simulink model "Sensor_Model"  (R2017b)
settings: Solver=VariableStepAuto  StartTime=0.0  StopTime=10.0  RelTol=1e-3
libraries: aerolibatmos2 x2
settings Model: Creator=pc  LastModifiedBy=pc

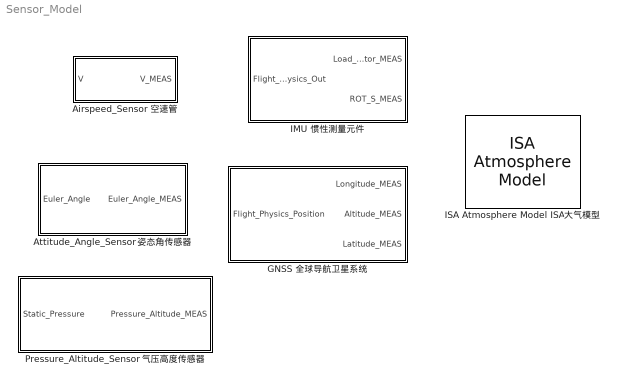
== system Sensor_Model ==
  Airspeed_Sensor 空速管 : Subsystem
  Attitude_Angle_Sensor 姿态角传感器 : Subsystem
  "GNSS 全球导航卫星系统 " : Subsystem
  IMU 惯性测量元件 : Subsystem
  ISA Atmosphere Model ISA大气模型 : aerolibatmos2/ISA Atmosphere Model  custom=off  g=9.80665  gamma=1.4  R=287.0531  L=0.0065  h_trop=11000  h_strat=20000  rho0=1.225  P0=101325  T0=288.15  h0=0
      settings: SourceProductName=Aerospace Blockset
  Pressure_Altitude_Sensor 气压高度传感器 : Subsystem

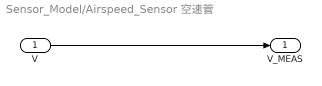
== system Sensor_Model/Airspeed_Sensor 空速管 ==
  V : Inport
  V_MEAS : Outport
  wires:
  V/1 -> V_MEAS/1

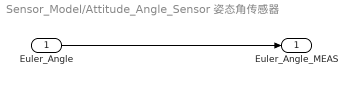
== system Sensor_Model/Attitude_Angle_Sensor 姿态角传感器 ==
  Euler_Angle : Inport
  Euler_Angle_MEAS : Outport
  wires:
  Euler_Angle/1 -> Euler_Angle_MEAS/1

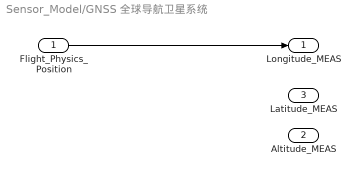
== system Sensor_Model/GNSS 全球导航卫星系统  ==
  Flight_Physics_Position : Inport
  Longitude_MEAS : Outport
  Altitude_MEAS : Outport  Port=2
  Latitude_MEAS : Outport  Port=3
  wires:
  Flight_Physics_Position/1 -> Longitude_MEAS/1

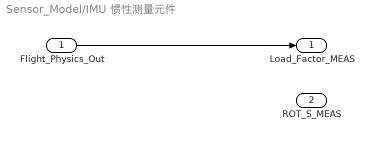
== system Sensor_Model/IMU 惯性测量元件 ==
  Flight_Physics_Out : Inport
  Load_Factor_MEAS : Outport
  ROT_S_MEAS : Outport  Port=2
  wires:
  Flight_Physics_Out/1 -> Load_Factor_MEAS/1

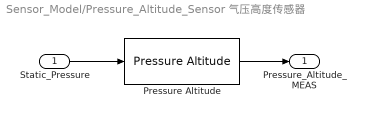
== system Sensor_Model/Pressure_Altitude_Sensor 气压高度传感器 ==
  Static_Pressure : Inport
  Pressure Altitude : aerolibatmos2/Pressure Altitude  units=Metric (MKS)  action=Warning
      settings: SourceProductName=Aerospace Blockset  SourceProductBaseCode=AE
  Pressure_Altitude_MEAS : Outport
  wires:
  Pressure Altitude/1 -> Pressure_Altitude_MEAS/1
  Static_Pressure/1 -> Pressure Altitude/1
